simulink model "CruiseControlSystem"  (R2024b)
settings: Solver=FixedStepAuto  StartTime=0.0  StopTime=15  FixedStep=SampleTime  RelTol=1e-3
model workspace (MAT data in the model file):
  SampleTime = 0.1
settings Model: Creator=MOHAMED  LastModifiedBy=MOHAMED

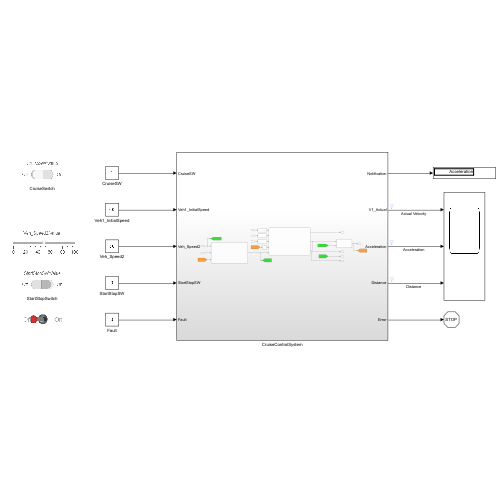
[thumbnail: Simulink's stored preview of the top-level diagram]
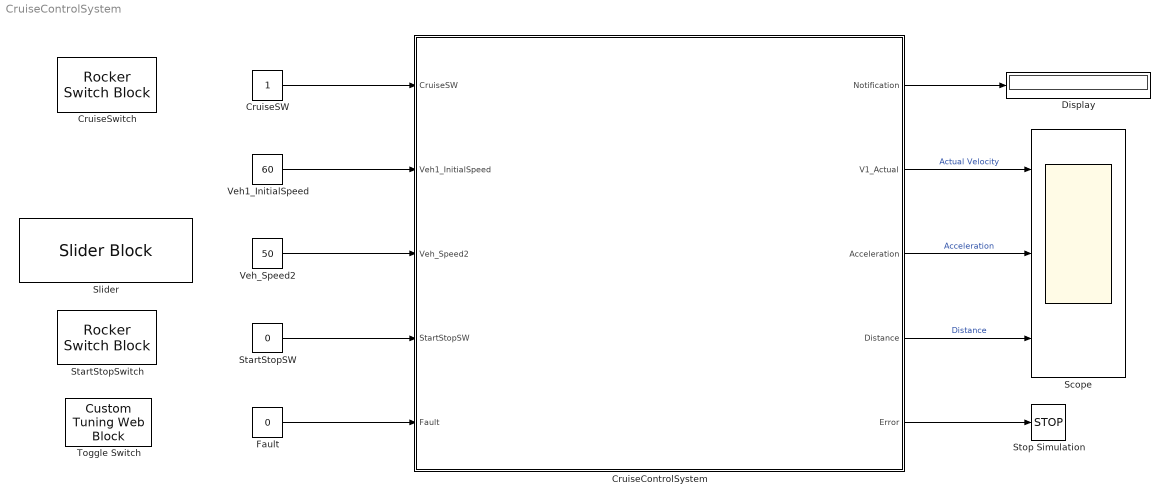
== system CruiseControlSystem ==
  CruiseControlSystem : Subsystem
  CruiseSW : Constant
  CruiseSwitch : RockerSwitchBlock
      settings: Values={{'Off', 'On'}, [0 1]}
  Display : Display
  Fault : Constant  Value=0
  Scope : Scope  NumInputPorts=3
  Slider : SliderBlock
  StartStopSW : Constant  Value=0
  StartStopSwitch : RockerSwitchBlock
      settings: Values={{'Off', 'On'}, [0 1]}
  Stop Simulation : Stop
  Toggle Switch : CustomTuningWebBlock  LabelPosition=Hide  ShowInitialText=on  Configuration="{\"components\":[{\"name\":\"CustomSwitchStateComponent\",\"settings\":{\"position\":[0,0,1,1],\"showAllLabels\":1,\"states\":[{\"HitRegion\":{\"position\":[0,0,0.5,1]},\"Image\":{\"position\":[0.24928571428571428,0,1,0.5014285714285714],\"size\":[1,0.5014285714285714],\"src\":\"data:image\\/svg+xml;base64,PHN2ZyB4bWxucz0iaHR0cDovL3d3dy53My5vcmcvMjAwMC9zdmciIHhtbG5zOnhsaW5rPSJodHRwOi8vd3d3LnczLm9yZy8xOTk5L3hsaW5rIiB2aWV3Qm94PSIwIDAgMzguMDQgMTUwIj48ZGVmcz48c3R5bGU+LmNscy0xe2ZpbGw6dXJsKCNyYWRpYWwtZ3JhZGllbnQpO30uY2xzLTJ7ZmlsbDp1cmwoI3JhZGlhbC1ncmFkaWVudC0yKTt9LmNscy0ze2ZpbGw6dXJsKCNXaGl0ZV9CbGFjayk7fS5jbHMtNHtmaWxsOnVybCgjcmFkaWFsLWdyYWRpZW50LTMpO30uY2xzLTV7ZmlsbDojNWI1YjViO30uY2xzLTZ7ZmlsbDp1cmwoI3Jh ...(+3556 chars)\",\"srcOrientation\":\"Right\"},\"Label\":{\"color\":[0.5019607843137255,0.5019607843137255,0.5019607843137255],\"icon\":{\"size\":[0,0],\"src\":[],\"srcOrientation\":\"Right\"},\"iconOffset\":0,\"iconPlacement\":\"left\",\"opacity\":1,\"position\":[0.5,0.07999999999999996],\"show\":true,\"text\":{\"content\":\"Off\",\"font\":\"Helvetica\"}},\"Value\":0},{\"HitRegion\":{\"position\":[0,0.5,0.5,1]},\"Image\":{\"position\":[0.24928571428571428,0,1,0.5014285714285714],\"size\":[1,0.5014285714285714],\"src\":\"data:image\\/svg+xml;base64,PHN2ZyB4bWxucz0iaHR0cDovL3d3dy53My5vcmcvMjAwMC9zdmciIHhtbG5zOnhsaW5rPSJodHRwOi8vd3d3LnczLm9yZy8xOTk5L3hsaW5rIiB2aWV3Qm94PSIwIDAgMzguMDQgMTUwIj48ZGVmcz48c3R5bGU+LmNscy0xe2ZpbGw6dXJsKCNyYWRpYWwtZ3JhZGllbnQpO30uY2xzLTJ7ZmlsbDp1cmwoI3JhZGlhbC1ncmFkaWVudC0yKTt9LmNscy0ze2ZpbGw6dXJsKCNXaGl0ZV9CbGFjayk7fS5jbHMtNHtmaWxsOnVybCgjcmFkaWFsLWdyYWRpZW50LTMpO30uY2xzLTV7ZmlsbDojNWI1YjViO30uY2xzLTZ7ZmlsbDp1cmwoI3Jh ...(+3628 chars)\",\"srcOrientation\":\"Right\"},\"Label\":{\"color\":[0.5019607843137255,0.5019607843137255,0.5019607843137255],\"icon\":{\"size\":[0,0],\"src\":[],\"srcOrientation\":\"Right\"},\"iconOffset\":0,\"iconPlacement\":\"left\",\"opacity\":1,\"position\":[0.5,0.92],\"show\":true,\"text\":{\"content\":\"On\",\"font\":\"Helvetica\"}},\"Value\":1}]}},{\"name\":\"BackgroundImageComponent\",\"settings\":{\"image\":{\"size\":[70,135],\"src\":\"default\",\"srcOrientation\":\"Right\"},\"position\":[0,0,1,1],\"scaleMode\":\"0\"}},{\"name\":\"ForegroundImageComponent\",\"settings\":{\"image\":{\"size\":[0,0],\"src\":\"default\",\"srcOrientation\":[]},\"isForeground\":1,\"position\":[0,0,1,1],\"scaleMode\":\"0\"}}],\"settings\":{\"BindingType\":\"param\",\"backgroundColor\":[0,0,0],\"backgroundOffset\":0.14,\"fixedAspectRatio\":\"on\",\"foregroundColor\":[0,0,0],\"showBackgroundColor\":false,\"variant\":\"toggle\",\"version\":\"R2024b\"},\"type\":\"Switch\"}"
  Veh1_InitialSpeed : Constant  Value=60
  Veh_Speed2 : Constant  Value=50
  wires:
  CruiseSW/1 -> CruiseControlSystem/1(CruiseSW)
  Veh1_InitialSpeed/1 -> CruiseControlSystem/2(Veh1_InitialSpeed)
  Veh_Speed2/1 -> CruiseControlSystem/3(Veh_Speed2)
  StartStopSW/1 -> CruiseControlSystem/4(StartStopSW)
  Fault/1 -> CruiseControlSystem/5(Fault)
  CruiseControlSystem/5(Error) -> Stop Simulation/1
  CruiseControlSystem/1(Notification) -> Display/1
  CruiseControlSystem/2(V1_Actual) -> Scope/1  "Actual Velocity"
  CruiseControlSystem/4(Distance) -> Scope/3  "Distance"
  CruiseControlSystem/3(Acceleration) -> Scope/2  "Acceleration"

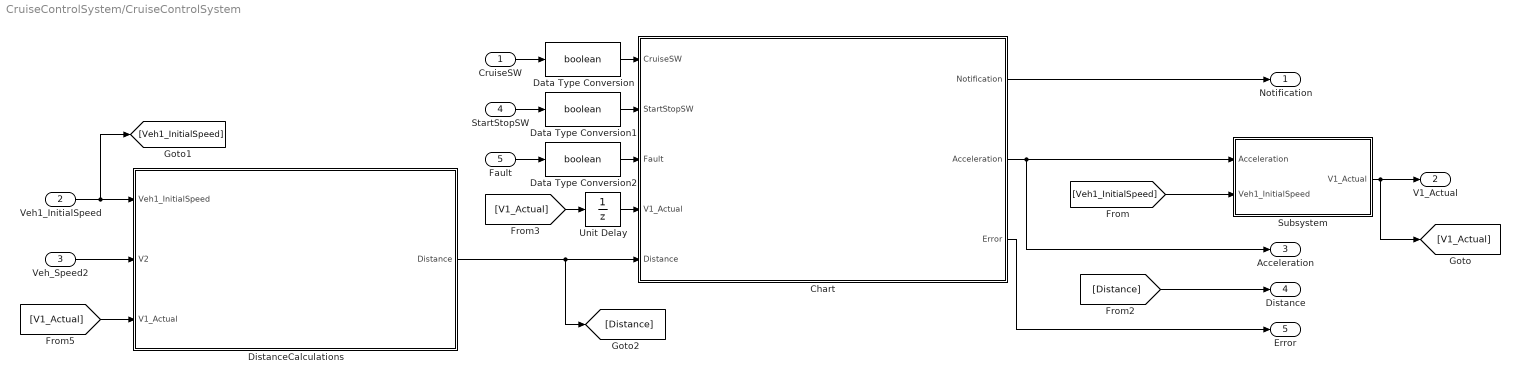
== system CruiseControlSystem/CruiseControlSystem ==
  CruiseSW : Inport
  Veh1_InitialSpeed : Inport  Port=2
  Veh_Speed2 : Inport  Port=3
  StartStopSW : Inport  Port=4
  Fault : Inport  Port=5
  Chart : Stateflow chart  TreatAsAtomicUnit=on
  Data Type Conversion : DataTypeConversion  OutDataTypeStr=boolean  SaturateOnIntegerOverflow=off  RndMeth=Floor
  Data Type Conversion1 : DataTypeConversion  OutDataTypeStr=boolean  SaturateOnIntegerOverflow=off  RndMeth=Floor
  Data Type Conversion2 : DataTypeConversion  OutDataTypeStr=boolean  SaturateOnIntegerOverflow=off  RndMeth=Floor
  DistanceCalculations : Subsystem
  Subsystem : Subsystem
  Unit Delay : UnitDelay  SampleTime=-1  HasFrameUpgradeWarning=on
  Notification : Outport
  V1_Actual : Outport  Port=2
  Acceleration : Outport  Port=3
  Distance : Outport  Port=4
  Error : Outport  Port=5
  wires:
  CruiseSW/1 -> Data Type Conversion/1
  Fault/1 -> Data Type Conversion2/1
  StartStopSW/1 -> Data Type Conversion1/1
  Veh1_InitialSpeed/1 -> [Veh1_InitialSpeed], DistanceCalculations/1(Veh1_InitialSpeed)
  Veh_Speed2/1 -> DistanceCalculations/2(V2)
  DistanceCalculations/1(Distance) -> [Distance], Chart/5(Distance)
  Chart/1(Notification) -> Notification/1
  Chart/3(Error) -> Error/1
  [Distance] -> Distance/1
  Data Type Conversion/1 -> Chart/1(CruiseSW)
  Data Type Conversion1/1 -> Chart/2(StartStopSW)
  Data Type Conversion2/1 -> Chart/3(Fault)
  [V1_Actual] -> Unit Delay/1
  Unit Delay/1 -> Chart/4(V1_Actual)
  Chart/2(Acceleration) -> Acceleration/1, Subsystem/1(Acceleration)
  [V1_Actual] -> DistanceCalculations/3(V1_Actual)
  Subsystem/1(V1_Actual) -> V1_Actual/1, [V1_Actual]
  [Veh1_InitialSpeed] -> Subsystem/2(Veh1_InitialSpeed)

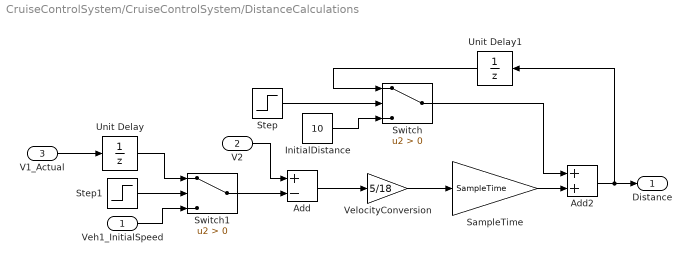
== system CruiseControlSystem/CruiseControlSystem/DistanceCalculations ==
  Veh1_InitialSpeed : Inport
  V2 : Inport  Port=2
  V1_Actual : Inport  Port=3
  Add : Sum  Inputs=+-
  Add2 : Sum
  InitialDistance : Constant  Value=10
  SampleTime : Gain  Gain=SampleTime
  Step : Step  Time=SampleTime  SampleTime=0
  Step1 : Step  Time=SampleTime  SampleTime=0
  Switch : Switch  Criteria=u2 > Threshold  SaturateOnIntegerOverflow=off  InputSameDT=off
  Switch1 : Switch  Criteria=u2 > Threshold  SaturateOnIntegerOverflow=off  InputSameDT=off
  Unit Delay : UnitDelay  SampleTime=SampleTime  HasFrameUpgradeWarning=on
  Unit Delay1 : UnitDelay  SampleTime=-1  HasFrameUpgradeWarning=on
  VelocityConversion : Gain  Gain=5/18
  Distance : Outport
  wires:
  V2/1 -> Add/1
  Veh1_InitialSpeed/1 -> Switch1/3
  Unit Delay/1 -> Switch1/1
  V1_Actual/1 -> Unit Delay/1
  Step1/1 -> Switch1/2
  Step/1 -> Switch/2
  InitialDistance/1 -> Switch/3
  Switch1/1 -> Add/2
  Switch/1 -> Add2/1
  Unit Delay1/1 -> Switch/1
  Add2/1 -> Distance/1, Unit Delay1/1
  VelocityConversion/1 -> SampleTime/1
  Add/1 -> VelocityConversion/1
  SampleTime/1 -> Add2/2

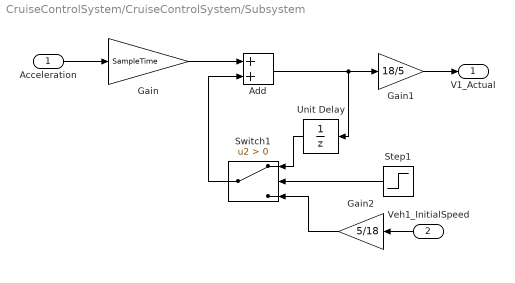
== system CruiseControlSystem/CruiseControlSystem/Subsystem ==
  Acceleration : Inport
  Veh1_InitialSpeed : Inport  Port=2
  Add : Sum
  Gain : Gain  Gain=SampleTime
  Gain1 : Gain  Gain=18/5
  Gain2 : Gain  Gain=5/18
  Step1 : Step  Time=SampleTime  SampleTime=0
  Switch1 : Switch  Criteria=u2 > Threshold  SaturateOnIntegerOverflow=off  InputSameDT=off
  Unit Delay : UnitDelay  SampleTime=-1  HasFrameUpgradeWarning=on
  V1_Actual : Outport
  wires:
  Acceleration/1 -> Gain/1
  Gain/1 -> Add/1
  Add/1 -> Unit Delay/1, Gain1/1
  Gain1/1 -> V1_Actual/1
  Step1/1 -> Switch1/2
  Unit Delay/1 -> Switch1/1
  Switch1/1 -> Add/2
  Veh1_InitialSpeed/1 -> Gain2/1
  Gain2/1 -> Switch1/3

== stateflow chart CruiseControlSystem/Chart ==
  state RegularState [parallel]
    settings: executionOrder=1
    state CruiseControlSystem_ON
      state Acceleration
        en, du:
        Notification = CarMode.Acceleration;
        Acceleration = 4;
      state Deceleration
        en, du:
        Notification = CarMode.Deceleration;
        Acceleration = -7;
      state Stop
        en, du:
        Flag = 1;
        Notification = CarMode.Stop;
        if(V1_Actual > 0)
        Acceleration = -15;
        else
        Acceleration = 0;
        end
      state Fault
        en:
        send(FaultOccured, FaultState);
        ex:
        send(FaultRemoved, FaultState);
      state DoNothing
        en:
        Notification = CarMode.DoNothing;
        Acceleration = 0;
      CruiseControlSystem_ON -> (junction 36) [order 1] : [Flag == 0]
      (junction 36) -> Acceleration [order 3] : [Distance > 15]
      (junction 36) -> Deceleration [order 4] : [Distance < 5]
      (junction 36) -> Stop [order 2] : [Distance < 1.5]
      (junction 36) -> Fault [order 1] : [Fault == 1]
      (junction 36) -> DoNothing [order 5] : [Distance > 5 && Distance < 10]
      (default) -> DoNothing
    state CruiseControlSystem_OFF
      en, du:
      Notification = CarMode.CruiseSystemOff;
    (default) -> CruiseControlSystem_ON
    CruiseControlSystem_ON -> CruiseControlSystem_OFF [order 1] : [CruiseSW == 0 || StartStopSW == 1]
    CruiseControlSystem_OFF -> CruiseControlSystem_ON : [CruiseSW == 1 && StartStopSW == 0]
  state FaultState [parallel]
    settings: executionOrder=2
    state Non_Fault_State
      en, du:
      Error = 0;
    state Non_Fault_State1
      en, du:
      Error = 1;
    (default) -> Non_Fault_State
    Non_Fault_State -> (junction 14) : FaultOccured{Notification = CarMode.FaultOccured}
    (junction 14) -> Non_Fault_State [order 1] : FaultRemoved
    (junction 14) -> Non_Fault_State1 [order 2] : after(5, sec)
  data: CruiseSW input; StartStopSW input; Fault input; V1_Actual input; Distance input; Notification output; Acceleration output double; Error output; Flag local double =0
  events: FaultOccured local FUNCTION_CALL_EVENT; FaultRemoved local FUNCTION_CALL_EVENT
